simulink model "hyd_hyb_2_opt_cont_test_new_1_col_ef_fin"  (Simulink 7.7)
settings: Solver=ode14x  StartTime=0  StopTime=530  FixedStep=0.01  MaxStep=.4  RelTol=1e-8
InitFcn:
  | const_3
values from neighbouring files (symbols this model uses):
  Af = 6.3    [brk_enrg.m]    (also in brk_enrg_1.m)
  BSFC_906_205 = [3.5684 4.3466 5.1668 6.0769 6.988 7.8992 8.8104 9.7336 10.8548 11.9809 13.1112 14.2571 ... (663 elements, 39x17)]    [BSFC_map_906_205.mat]
  Cd = 0.55    [brk_enrg.m]    (also in brk_enrg_1.m)
  den = 1.202    [brk_enrg.m]    (also in brk_enrg_1.m)
  fr = 0.01    [brk_enrg.m]    (also in brk_enrg_1.m)
undefined symbols (not defined in the file or in its folder): clutchRise, down_spd_2, down_spd_3, down_spd_4, down_spd_c, fuel_density, gearshift, I_wheel, Idle_spd_eng_906, M1_hydr, p_v_15, pmax_125, qv_125, Rw, sec_eng_sfc_map, T_max_906, T_min, TC_spd_ratio_max, torque_convertor, Twait, up_spd_1, up_spd_2, up_spd_3, up_spd_c, v_p_10, v_p_15, v_p_5
libraries: neural x327, fl_lib x43, nesl_utility x30, sdl_lib x14, simulink x4, simulink_need_slupdate x1
(part 3 of 10)

== system hyd_hyb_2_opt_cont_test_new_1_col_ef_fin/Transmission1/Torque Convertor/main solver/Torque generation ==
  note: TORQUE CONVERTER
  note: Not motoring mode is neglected
  Turbine speed (rad/s) : Inport
  Impeller speed (rad/s) : Inport  Port=2
  4 : Product  Inputs=/*  SaturateOnIntegerOverflow=on  RndMeth=Zero  InputSameDT=on  OutDataTypeStr=Inherit: Same as first input
  Constant1 : Constant
  Constant2 : Constant  Value=eps
  Constant6 : Constant  Value=TC_spd_ratio_max
  Gain1 : Gain  Gain=-1  SaturateOnIntegerOverflow=on  OutDataTypeStr=Inherit: Same as input  ParamDataTypeStr=Inherit: Same as input
  Math Function1 : Math  Operator=square  SaturateOnIntegerOverflow=on
  Memory : Memory
  Memory1 : Memory
  MinMax2 : MinMax  Function=max  Inputs=2  ZeroCross=off
  Mu : Lookup  InputValues=torque_convertor(:,1)  Table=torque_convertor(:,2)  SaturateOnIntegerOverflow=on
  Ref_spd (rpm) : Constant  Value=1000
  T1 : Scope  NumInputPorts=2
      settings: YMin=75~-5  YMax=165~5  SaveName=ScopeData19
  T_i : Product  Inputs=**  SaturateOnIntegerOverflow=on  RndMeth=Zero  InputSameDT=on  OutDataTypeStr=Inherit: Same as first input
  T_t : Product  Inputs=**  SaturateOnIntegerOverflow=on  RndMeth=Zero  InputSameDT=on  OutDataTypeStr=Inherit: Same as first input
  check pump spd=0 : Switch  Threshold=0.1
  check turb spd=0 : Switch  Threshold=0.1
  pump T : Lookup  InputValues=torque_convertor(:,1)  Table=torque_convertor(:,3)  SaturateOnIntegerOverflow=on
  rad/s 2 rpm : Gain  Gain=60/(2*pi)
  speed ratio : Product  Inputs=/*  SaturateOnIntegerOverflow=on  RndMeth=Zero  InputSameDT=on  OutDataTypeStr=Inherit: Same as first input
  Turbine torque : Outport
  Impeller torque : Outport  Port=2
  wires:
  Constant2/1 -> MinMax2/2
  MinMax2/1 -> speed ratio/1
  Impeller speed (rad/s)/1 -> MinMax2/1, check pump spd=0/2, rad/s 2 rpm/1
  Turbine speed (rad/s)/1 -> check turb spd=0/2, speed ratio/2
  speed ratio/1 -> check pump spd=0/1
  Constant1/1 -> check turb spd=0/3
  Constant6/1 -> check turb spd=0/1
  check turb spd=0/1 -> check pump spd=0/3
  check pump spd=0/1 -> Mu/1, pump T/1
  Ref_spd (rpm)/1 -> 4/1
  rad/s 2 rpm/1 -> 4/2
  4/1 -> Math Function1/1
  pump T/1 -> T_i/1
  Math Function1/1 -> T_i/2
  T_i/1 -> T_t/2, Gain1/1
  Gain1/1 -> Memory1/1
  Mu/1 -> T_t/1
  T_t/1 -> Memory/1
  Memory/1 -> Turbine torque/1
  Memory1/1 -> Impeller torque/1

== system hyd_hyb_2_opt_cont_test_new_1_col_ef_fin/Transmission1/gear box/gear box/Clutch Control ==
  control : Inport
  1 : Constant
  2 : Constant  Value=2
  3 : Constant  Value=3
  4 : Constant  Value=4
  Add{,1..3} (4 alike) : Sum  Inputs=+-
  Enabled Subsystem1 : Subsystem  TreatAsAtomicUnit=on
  Enabled Subsystem2 : Subsystem  TreatAsAtomicUnit=on
  Enabled Subsystem3 : Subsystem  TreatAsAtomicUnit=on
  Enabled Subsystem4 : Subsystem  TreatAsAtomicUnit=on
  Mux2 : Mux
  disengahe : Constant  Value=-1
  engage : Constant
  selector{1..4} (4 alike) : Switch  Criteria=u2 ~= 0  Threshold=2300  ZeroCross=off
  Clutches : Outport
  wires:
  Mux2/1 -> Clutches/1
  engage/1 -> [engage]
  [disengage] -> selector1/1
  disengahe/1 -> [disengage]
  [engage] -> selector1/3
  control/1 -> Add/1, Add1/1, Add2/1, Add3/1
  Add/1 -> selector1/2
  1/1 -> Add/2
  [disengage] -> selector2/1
  [engage] -> selector2/3
  Add1/1 -> selector2/2
  2/1 -> Add1/2
  [disengage] -> selector3/1
  [engage] -> selector3/3
  Add2/1 -> selector3/2
  3/1 -> Add2/2
  [disengage] -> selector4/1
  [engage] -> selector4/3
  Add3/1 -> selector4/2
  4/1 -> Add3/2
  selector1/1 -> Enabled Subsystem1/Enable
  selector2/1 -> Enabled Subsystem2/Enable
  selector3/1 -> Enabled Subsystem3/Enable
  selector4/1 -> Enabled Subsystem4/Enable
  Enabled Subsystem1/1(clutch release) -> Mux2/1
  Enabled Subsystem2/1(clutch release) -> Mux2/2
  Enabled Subsystem3/1(clutch release) -> Mux2/3
  Enabled Subsystem4/1(clutch release) -> Mux2/4

== system hyd_hyb_2_opt_cont_test_new_1_col_ef_fin/controller1/optimized controller - pm/net_col_ef_1/Layer 1 ==
  "p{1}" : Inport  PortDimensions=3
      mask Display: e = 0.06;c1 = [120 230 180]/255;c2 = ([120 230 180]+0)/(256+128);c3 = ([120 230 180]+128)/(256+128);patch([0 1 1 0],[0 0 1 1],c1);patch([0 1 1 1-e 1-e 0+e],[0 0 1 1-e 0+e 0+e],c2);patch([0 0 1 1-e 0+e 0+e],[0 1 1 1-e 1-e 0+e],c3);plot([0 1 1 0 0],[0 0 1 1 0]);
  Delays 1 : Subsystem
      mask Display: e = 0.06;c1 = [120 150 230]/255;c2 = ([120 150 230]+0)/383;c3 = ([120 150 230]+128)/383;patch([0 1 1 0],[0 0 1 1],c1);patch([0 1 1 1-e 1-e 0+e],[0 0 1 1-e 0+e 0+e],c2);patch([0 0 1 1-e 0+e 0+e],[0 1 1 1-e 1-e 0+e],c3);plot([0 1 1 0 0],[0 0 1 1 0]);disp('0');
  "IW{1,1}" : Subsystem
      mask Display: e = 0.06;c1 = [120 150 230]/255;c2 = ([120 150 230]+0)/383;c3 = ([120 150 230]+128)/383;patch([0 1 1 0],[0 0 1 1],c1);patch([0 1 1 1-e 1-e 0+e],[0 0 1 1-e 0+e 0+e],c2);patch([0 0 1 1-e 0+e 0+e],[0 1 1 1-e 1-e 0+e],c3);plot([0 1 1 0 0],[0 0 1 1 0]);disp('W');
  "b{1}" : Constant  Value=[10.272884338164415;10.158388839610668;-8.8137585907009761;-8.6570271257242233;-8.8970383233546322;-8.3732297223932406;-8.2902058826026686;-8.3765329651302221;-8.1601725859937311;7.3878677135191477;5.9137474143171671;6.0189008328843263;-4.7198199500370155;-4.5492439595817009;-3.6590612602413786;-4.0868738376274472;-3.2611974200680032;-2.5669983522012405;2.8521134680955162;-1.9645715433960607;-2.0075702387778405;-2.2689062882637798;1.7944973393296622;-0.60777657516365402;-0.33335423588948843;0.70492263184083259;1.0038561719860595;0.8312957719409716;2.0241730304275114;2.4288729886427602;-1.5051652534112119;-2.9602742871001562;3.5101998859041661;4.4839700583582864;-5.3527641027608928;4.8621496598397966;-4.4065527200098753;5.333150061440934;5.4587754651459868;6.0824002270216777;6.163842184650008;6.5644779762447678;7.0617890841349729;7.5844337833421029;-8.3589611799416907;9.2543399894272227;9.1887230177194503;-8.8917972218632144;10.192523469036553;-10.477571329366949]
      mask Display: e = 0.06;c1 = [120 150 230]/255;c2 = ([120 150 230]+0)/383;c3 = ([120 150 230]+128)/383;patch([0 1 1 0],[0 0 1 1],c1);patch([0 1 1 1-e 1-e 0+e],[0 0 1 1-e 0+e 0+e],c2);patch([0 0 1 1-e 0+e 0+e],[0 1 1 1-e 1-e 0+e],c3);plot([0 1 1 0 0],[0 0 1 1 0]);disp('b');
  logsig : neural/Transfer Functions/logsig  SystemSampleTime=-1
  netsum : Sum  Inputs=2  SaturateOnIntegerOverflow=on  InputSameDT=on  OutDataTypeStr=Inherit: Same as first input
      mask Display: e = 0.06;c1 = [120 150 230]/255;c2 = ([120 150 230]+0)/383;c3 = ([120 150 230]+128)/383;patch([0 1 1 0],[0 0 1 1],c1);patch([0 1 1 1-e 1-e 0+e],[0 0 1 1-e 0+e 0+e],c2);patch([0 0 1 1-e 0+e 0+e],[0 1 1 1-e 1-e 0+e],c3);plot([0 1 1 0 0],[0 0 1 1 0]);disp('+');
  "a{1}" : Outport  InitialOutput=[0;0;0;0;0;0;0;0;0;0;0;0;0;0;0;0;0;0;0;0;0;0;0;0;0;0;0;0;0;0;0;0;0;0;0;0;0;0;0;0;0;0;0;0;0;0;0;0;0;0]
      mask Display: e = 0.06;c1 = [120 230 180]/255;c2 = ([120 230 180]+0)/(256+128);c3 = ([120 230 180]+128)/(256+128);patch([0 1 1 0],[0 0 1 1],c1);patch([0 1 1 1-e 1-e 0+e],[0 0 1 1-e 0+e 0+e],c2);patch([0 0 1 1-e 0+e 0+e],[0 1 1 1-e 1-e 0+e],c3);plot([0 1 1 0 0],[0 0 1 1 0]);
  wires:
  "p{1}"/1 -> Delays 1/1("p{1}")
  Delays 1/1("pd{1,1}") -> "IW{1,1}"/1("pd{1,1}")
  "IW{1,1}"/1("iz{1,1}") -> netsum/1
  "b{1}"/1 -> netsum/2
  netsum/1 -> logsig/1
  logsig/1 -> "a{1}"/1

== system hyd_hyb_2_opt_cont_test_new_1_col_ef_fin/controller1/optimized controller - pm/net_col_ef_1/Layer 2 ==
  "a{1} " : Inport  PortDimensions=50
      mask Display: e = 0.06;c1 = [120 230 180]/255;c2 = ([120 230 180]+0)/(256+128);c3 = ([120 230 180]+128)/(256+128);patch([0 1 1 0],[0 0 1 1],c1);patch([0 1 1 1-e 1-e 0+e],[0 0 1 1-e 0+e 0+e],c2);patch([0 0 1 1-e 0+e 0+e],[0 1 1 1-e 1-e 0+e],c3);plot([0 1 1 0 0],[0 0 1 1 0]);
  Delays 1 : Subsystem
      mask Display: e = 0.06;c1 = [120 150 230]/255;c2 = ([120 150 230]+0)/383;c3 = ([120 150 230]+128)/383;patch([0 1 1 0],[0 0 1 1],c1);patch([0 1 1 1-e 1-e 0+e],[0 0 1 1-e 0+e 0+e],c2);patch([0 0 1 1-e 0+e 0+e],[0 1 1 1-e 1-e 0+e],c3);plot([0 1 1 0 0],[0 0 1 1 0]);disp('0');
  "LW{2,1}" : Subsystem
      mask Display: e = 0.06;c1 = [120 150 230]/255;c2 = ([120 150 230]+0)/383;c3 = ([120 150 230]+128)/383;patch([0 1 1 0],[0 0 1 1],c1);patch([0 1 1 1-e 1-e 0+e],[0 0 1 1-e 0+e 0+e],c2);patch([0 0 1 1-e 0+e 0+e],[0 1 1 1-e 1-e 0+e],c3);plot([0 1 1 0 0],[0 0 1 1 0]);disp('W');
  "b{2}" : Constant  Value=[-1.4746968992061404;6.761460429459289;4.8593062407264256;-2.4434548501711921;2.8014335830561317;-1.2377617866407475;0.60970112347272343;6.0004453403634397;1.5023634362208427;-2.3253426322313246;-5.3357671798553792;2.2138042378012139;-3.2204621848726322;-0.91358517604309897;-4.265772269140677;-0.49547425424668967;2.7481974655284684;2.6522900082012191;-1.450078084740686;5.9357949258451921;-1.1096734624746596;-1.9216781485245211;1.5013570287327187;-3.1725593392467553;0.070873309951381178;1.4583370245475129;-1.380987170740555;-4.9014727609251594;-2.421891114631245;-0.045879446762915062;2.3447338445340051;5.0580315597432879;2.2792762573025591;4.0979703997466634;-0.41868820623327574;0.59156567080418943;1.93176393811276;3.5095523399155435;-3.5434554285500419;3.8577559424144559;0.1840496036646519;0.80556867719655356;-2.1746365989617589;1.7602851911002209;-0.17757596753320681;5.9726215463790888;-4.0530999585525285;4.0472988103686962;7.3387320715217763;-0.86522529377217905]
      mask Display: e = 0.06;c1 = [120 150 230]/255;c2 = ([120 150 230]+0)/383;c3 = ([120 150 230]+128)/383;patch([0 1 1 0],[0 0 1 1],c1);patch([0 1 1 1-e 1-e 0+e],[0 0 1 1-e 0+e 0+e],c2);patch([0 0 1 1-e 0+e 0+e],[0 1 1 1-e 1-e 0+e],c3);plot([0 1 1 0 0],[0 0 1 1 0]);disp('b');
  logsig : neural/Transfer Functions/logsig  SystemSampleTime=-1
  netsum : Sum  Inputs=2  SaturateOnIntegerOverflow=on  InputSameDT=on  OutDataTypeStr=Inherit: Same as first input
      mask Display: e = 0.06;c1 = [120 150 230]/255;c2 = ([120 150 230]+0)/383;c3 = ([120 150 230]+128)/383;patch([0 1 1 0],[0 0 1 1],c1);patch([0 1 1 1-e 1-e 0+e],[0 0 1 1-e 0+e 0+e],c2);patch([0 0 1 1-e 0+e 0+e],[0 1 1 1-e 1-e 0+e],c3);plot([0 1 1 0 0],[0 0 1 1 0]);disp('+');
  "a{2}" : Outport  InitialOutput=[0;0;0;0;0;0;0;0;0;0;0;0;0;0;0;0;0;0;0;0;0;0;0;0;0;0;0;0;0;0;0;0;0;0;0;0;0;0;0;0;0;0;0;0;0;0;0;0;0;0]
      mask Display: e = 0.06;c1 = [120 230 180]/255;c2 = ([120 230 180]+0)/(256+128);c3 = ([120 230 180]+128)/(256+128);patch([0 1 1 0],[0 0 1 1],c1);patch([0 1 1 1-e 1-e 0+e],[0 0 1 1-e 0+e 0+e],c2);patch([0 0 1 1-e 0+e 0+e],[0 1 1 1-e 1-e 0+e],c3);plot([0 1 1 0 0],[0 0 1 1 0]);
  wires:
  "a{1} "/1 -> Delays 1/1("p{2}")
  Delays 1/1("pd{2,1}") -> "LW{2,1}"/1("ad{2,1}")
  "LW{2,1}"/1("lz{2,1}") -> netsum/1
  "b{2}"/1 -> netsum/2
  netsum/1 -> logsig/1
  logsig/1 -> "a{2}"/1

== system hyd_hyb_2_opt_cont_test_new_1_col_ef_fin/controller1/optimized controller - pm/net_col_ef_1/Layer 3 ==
  "a{2} " : Inport  PortDimensions=50
      mask Display: e = 0.06;c1 = [120 230 180]/255;c2 = ([120 230 180]+0)/(256+128);c3 = ([120 230 180]+128)/(256+128);patch([0 1 1 0],[0 0 1 1],c1);patch([0 1 1 1-e 1-e 0+e],[0 0 1 1-e 0+e 0+e],c2);patch([0 0 1 1-e 0+e 0+e],[0 1 1 1-e 1-e 0+e],c3);plot([0 1 1 0 0],[0 0 1 1 0]);
  Delays 1 : Subsystem
      mask Display: e = 0.06;c1 = [120 150 230]/255;c2 = ([120 150 230]+0)/383;c3 = ([120 150 230]+128)/383;patch([0 1 1 0],[0 0 1 1],c1);patch([0 1 1 1-e 1-e 0+e],[0 0 1 1-e 0+e 0+e],c2);patch([0 0 1 1-e 0+e 0+e],[0 1 1 1-e 1-e 0+e],c3);plot([0 1 1 0 0],[0 0 1 1 0]);disp('0');
  "LW{3,2}" : Subsystem
      mask Display: e = 0.06;c1 = [120 150 230]/255;c2 = ([120 150 230]+0)/383;c3 = ([120 150 230]+128)/383;patch([0 1 1 0],[0 0 1 1],c1);patch([0 1 1 1-e 1-e 0+e],[0 0 1 1-e 0+e 0+e],c2);patch([0 0 1 1-e 0+e 0+e],[0 1 1 1-e 1-e 0+e],c3);plot([0 1 1 0 0],[0 0 1 1 0]);disp('W');
  "b{3}" : Constant  Value=-0.53255115865547076
      mask Display: e = 0.06;c1 = [120 150 230]/255;c2 = ([120 150 230]+0)/383;c3 = ([120 150 230]+128)/383;patch([0 1 1 0],[0 0 1 1],c1);patch([0 1 1 1-e 1-e 0+e],[0 0 1 1-e 0+e 0+e],c2);patch([0 0 1 1-e 0+e 0+e],[0 1 1 1-e 1-e 0+e],c3);plot([0 1 1 0 0],[0 0 1 1 0]);disp('b');
  netsum : Sum  Inputs=2  SaturateOnIntegerOverflow=on  InputSameDT=on  OutDataTypeStr=Inherit: Same as first input
      mask Display: e = 0.06;c1 = [120 150 230]/255;c2 = ([120 150 230]+0)/383;c3 = ([120 150 230]+128)/383;patch([0 1 1 0],[0 0 1 1],c1);patch([0 1 1 1-e 1-e 0+e],[0 0 1 1-e 0+e 0+e],c2);patch([0 0 1 1-e 0+e 0+e],[0 1 1 1-e 1-e 0+e],c3);plot([0 1 1 0 0],[0 0 1 1 0]);disp('+');
  purelin : neural/Transfer Functions/purelin  SystemSampleTime=-1
  "a{3}" : Outport  InitialOutput=0
      mask Display: e = 0.06;c1 = [120 230 180]/255;c2 = ([120 230 180]+0)/(256+128);c3 = ([120 230 180]+128)/(256+128);patch([0 1 1 0],[0 0 1 1],c1);patch([0 1 1 1-e 1-e 0+e],[0 0 1 1-e 0+e 0+e],c2);patch([0 0 1 1-e 0+e 0+e],[0 1 1 1-e 1-e 0+e],c3);plot([0 1 1 0 0],[0 0 1 1 0]);
  wires:
  "a{2} "/1 -> Delays 1/1("p{3}")
  Delays 1/1("pd{3,2}") -> "LW{3,2}"/1("ad{3,2}")
  "LW{3,2}"/1("lz{3,2}") -> netsum/1
  "b{3}"/1 -> netsum/2
  netsum/1 -> purelin/1
  purelin/1 -> "a{3}"/1

== system hyd_hyb_2_opt_cont_test_new_1_col_ef_fin/controller1/optimized controller - pm/net_col_ef_1/Process Input 1 ==
  x : Inport  PortDimensions=3
      mask Display: e = 0.06;c1 = [120 230 180]/255;c2 = ([120 230 180]+0)/(256+128);c3 = ([120 230 180]+128)/(256+128);patch([0 1 1 0],[0 0 1 1],c1);patch([0 1 1 1-e 1-e 0+e],[0 0 1 1-e 0+e 0+e],c2);patch([0 0 1 1-e 0+e 0+e],[0 1 1 1-e 1-e 0+e],c3);plot([0 1 1 0 0],[0 0 1 1 0]);
  fixunknowns : neural/Processing Functions/fixunknowns  SystemSampleTime=-1  inputSize=3  indices=[1 2 3]
  mapminmax : neural/Processing Functions/mapminmax  SystemSampleTime=-1  xmin=[0;0;0]  xmax=[0.90000000000000013;1.009090909090909;0.63716399999999995]  ymin=-1  ymax=1
  removeconstantrows : neural/Processing Functions/removeconstantrows  SystemSampleTime=-1  inputSize=3  keep=[1 2 3]
  p : Outport  PortDimensions=3
      mask Display: e = 0.06;c1 = [120 230 180]/255;c2 = ([120 230 180]+0)/(256+128);c3 = ([120 230 180]+128)/(256+128);patch([0 1 1 0],[0 0 1 1],c1);patch([0 1 1 1-e 1-e 0+e],[0 0 1 1-e 0+e 0+e],c2);patch([0 0 1 1-e 0+e 0+e],[0 1 1 1-e 1-e 0+e],c3);plot([0 1 1 0 0],[0 0 1 1 0]);
  wires:
  x/1 -> fixunknowns/1
  fixunknowns/1 -> removeconstantrows/1
  removeconstantrows/1 -> mapminmax/1
  mapminmax/1 -> p/1

== system hyd_hyb_2_opt_cont_test_new_1_col_ef_fin/controller1/optimized controller - pm/net_col_ef_1/Process Output 1 ==
  a : Inport  PortDimensions=1
      mask Display: e = 0.06;c1 = [120 230 180]/255;c2 = ([120 230 180]+0)/(256+128);c3 = ([120 230 180]+128)/(256+128);patch([0 1 1 0],[0 0 1 1],c1);patch([0 1 1 1-e 1-e 0+e],[0 0 1 1-e 0+e 0+e],c2);patch([0 0 1 1-e 0+e 0+e],[0 1 1 1-e 1-e 0+e],c3);plot([0 1 1 0 0],[0 0 1 1 0]);
  mapminmax_reverse : neural/Processing Functions/mapminmax_reverse  SystemSampleTime=-1  xmin=0  xmax=0.9015181489837879  ymin=-1  ymax=1
  removeconstantrows_reverse : neural/Processing Functions/removeconstantrows_reverse  SystemSampleTime=-1  inputSize=1  constants=zeros(0,1)  rearrange=1
  y : Outport  PortDimensions=1
      mask Display: e = 0.06;c1 = [120 230 180]/255;c2 = ([120 230 180]+0)/(256+128);c3 = ([120 230 180]+128)/(256+128);patch([0 1 1 0],[0 0 1 1],c1);patch([0 1 1 1-e 1-e 0+e],[0 0 1 1-e 0+e 0+e],c2);patch([0 0 1 1-e 0+e 0+e],[0 1 1 1-e 1-e 0+e],c3);plot([0 1 1 0 0],[0 0 1 1 0]);
  wires:
  a/1 -> mapminmax_reverse/1
  mapminmax_reverse/1 -> removeconstantrows_reverse/1
  removeconstantrows_reverse/1 -> y/1

== system hyd_hyb_2_opt_cont_test_new_1_col_ef_fin/controller1/optimized controller - pm/net_col_ef_2/Layer 1 ==
  "p{1}" : Inport  PortDimensions=3
      mask Display: e = 0.06;c1 = [120 230 180]/255;c2 = ([120 230 180]+0)/(256+128);c3 = ([120 230 180]+128)/(256+128);patch([0 1 1 0],[0 0 1 1],c1);patch([0 1 1 1-e 1-e 0+e],[0 0 1 1-e 0+e 0+e],c2);patch([0 0 1 1-e 0+e 0+e],[0 1 1 1-e 1-e 0+e],c3);plot([0 1 1 0 0],[0 0 1 1 0]);
  Delays 1 : Subsystem
      mask Display: e = 0.06;c1 = [120 150 230]/255;c2 = ([120 150 230]+0)/383;c3 = ([120 150 230]+128)/383;patch([0 1 1 0],[0 0 1 1],c1);patch([0 1 1 1-e 1-e 0+e],[0 0 1 1-e 0+e 0+e],c2);patch([0 0 1 1-e 0+e 0+e],[0 1 1 1-e 1-e 0+e],c3);plot([0 1 1 0 0],[0 0 1 1 0]);disp('0');
  "IW{1,1}" : Subsystem
      mask Display: e = 0.06;c1 = [120 150 230]/255;c2 = ([120 150 230]+0)/383;c3 = ([120 150 230]+128)/383;patch([0 1 1 0],[0 0 1 1],c1);patch([0 1 1 1-e 1-e 0+e],[0 0 1 1-e 0+e 0+e],c2);patch([0 0 1 1-e 0+e 0+e],[0 1 1 1-e 1-e 0+e],c3);plot([0 1 1 0 0],[0 0 1 1 0]);disp('W');
  "b{1}" : Constant  Value=[11.06291160506464;9.6569498895400336;9.7057218735701358;9.3112833261288372;8.7376413828696577;7.5818969929168896;-7.689186662963075;6.8841555682455375;5.480543380122934;-6.7353338753925431;-6.2439434769565203;-4.7494739295836874;-4.95737643411577;-4.6437259198738037;3.5304849746771545;-4.1757390830539922;-3.0584729883330146;-3.1420690410497674;-2.7312479968531616;-2.761085247415719;0.94765649190303802;1.1617110605498155;0.97691124339635782;0.79251198170241977;0.20894216666912813;-0.89968169007623477;-0.5079308913259809;-1.1247392235072682;1.7484351351117244;-1.7461420332640352;-2.3679372815024879;-2.4585499737006038;4.5049715514684214;3.7433756567561591;4.3924005740068113;-4.4562245200249722;4.5180694005112034;-5.3308269964363113;5.9176445995746247;-6.1338393655658079;-6.5153465860809519;-6.9387105180769808;8.3926806026615441;-7.8456184342767861;8.170511983096354;8.7628634893332684;-9.0774508782222547;-8.537231421878209;-9.8218508072603683;9.9868721404365726]
      mask Display: e = 0.06;c1 = [120 150 230]/255;c2 = ([120 150 230]+0)/383;c3 = ([120 150 230]+128)/383;patch([0 1 1 0],[0 0 1 1],c1);patch([0 1 1 1-e 1-e 0+e],[0 0 1 1-e 0+e 0+e],c2);patch([0 0 1 1-e 0+e 0+e],[0 1 1 1-e 1-e 0+e],c3);plot([0 1 1 0 0],[0 0 1 1 0]);disp('b');
  logsig : neural/Transfer Functions/logsig  SystemSampleTime=-1
  netsum : Sum  Inputs=2  SaturateOnIntegerOverflow=on  InputSameDT=on  OutDataTypeStr=Inherit: Same as first input
      mask Display: e = 0.06;c1 = [120 150 230]/255;c2 = ([120 150 230]+0)/383;c3 = ([120 150 230]+128)/383;patch([0 1 1 0],[0 0 1 1],c1);patch([0 1 1 1-e 1-e 0+e],[0 0 1 1-e 0+e 0+e],c2);patch([0 0 1 1-e 0+e 0+e],[0 1 1 1-e 1-e 0+e],c3);plot([0 1 1 0 0],[0 0 1 1 0]);disp('+');
  "a{1}" : Outport  InitialOutput=[0;0;0;0;0;0;0;0;0;0;0;0;0;0;0;0;0;0;0;0;0;0;0;0;0;0;0;0;0;0;0;0;0;0;0;0;0;0;0;0;0;0;0;0;0;0;0;0;0;0]
      mask Display: e = 0.06;c1 = [120 230 180]/255;c2 = ([120 230 180]+0)/(256+128);c3 = ([120 230 180]+128)/(256+128);patch([0 1 1 0],[0 0 1 1],c1);patch([0 1 1 1-e 1-e 0+e],[0 0 1 1-e 0+e 0+e],c2);patch([0 0 1 1-e 0+e 0+e],[0 1 1 1-e 1-e 0+e],c3);plot([0 1 1 0 0],[0 0 1 1 0]);
  wires:
  "p{1}"/1 -> Delays 1/1("p{1}")
  Delays 1/1("pd{1,1}") -> "IW{1,1}"/1("pd{1,1}")
  "IW{1,1}"/1("iz{1,1}") -> netsum/1
  "b{1}"/1 -> netsum/2
  netsum/1 -> logsig/1
  logsig/1 -> "a{1}"/1

== system hyd_hyb_2_opt_cont_test_new_1_col_ef_fin/controller1/optimized controller - pm/net_col_ef_2/Layer 2 ==
  "a{1} " : Inport  PortDimensions=50
      mask Display: e = 0.06;c1 = [120 230 180]/255;c2 = ([120 230 180]+0)/(256+128);c3 = ([120 230 180]+128)/(256+128);patch([0 1 1 0],[0 0 1 1],c1);patch([0 1 1 1-e 1-e 0+e],[0 0 1 1-e 0+e 0+e],c2);patch([0 0 1 1-e 0+e 0+e],[0 1 1 1-e 1-e 0+e],c3);plot([0 1 1 0 0],[0 0 1 1 0]);
  Delays 1 : Subsystem
      mask Display: e = 0.06;c1 = [120 150 230]/255;c2 = ([120 150 230]+0)/383;c3 = ([120 150 230]+128)/383;patch([0 1 1 0],[0 0 1 1],c1);patch([0 1 1 1-e 1-e 0+e],[0 0 1 1-e 0+e 0+e],c2);patch([0 0 1 1-e 0+e 0+e],[0 1 1 1-e 1-e 0+e],c3);plot([0 1 1 0 0],[0 0 1 1 0]);disp('0');
  "LW{2,1}" : Subsystem
      mask Display: e = 0.06;c1 = [120 150 230]/255;c2 = ([120 150 230]+0)/383;c3 = ([120 150 230]+128)/383;patch([0 1 1 0],[0 0 1 1],c1);patch([0 1 1 1-e 1-e 0+e],[0 0 1 1-e 0+e 0+e],c2);patch([0 0 1 1-e 0+e 0+e],[0 1 1 1-e 1-e 0+e],c3);plot([0 1 1 0 0],[0 0 1 1 0]);disp('W');
  "b{2}" : Constant  Value=[1.2957023881188001;-8.4250423006678865;-0.83849144117593744;5.1940231045960283;-2.8277581624328021;2.323521888729871;-0.47657758453361571;-1.4935523337583885;6.2630674201555294;3.9356633739489526;-3.3711843755045723;-0.91849200872177161;2.3155313979295107;5.2316800014222249;-1.549962088505253;2.6578906811948371;-4.0210651554100005;1.1726109689860429;-3.5551891275712766;-0.63513021573007333;0.78168202695753253;-2.5466977416139245;-3.1494465602922777;4.5806898083337355;7.8804370668016537;2.0015927562451705;4.4640169205076878;-0.85047345033081234;4.2406992651338431;-4.5935384604573288;-3.278093976124933;-4.5782806163281355;-1.363012863764252;-0.91938331656109173;-4.9024295612468514;0.8809270622210823;-0.66333942549327818;-0.49112451411523284;-5.6624444398120888;-0.84647761333632732;-2.5444084615881972;-8.0610468494463348;0.61998104669407039;-4.5620258732554246;0.45894670318714587;1.1974781726729835;2.2804204429841644;0.38514422559041417;2.8834613502054052;-0.82401605208817619]
      mask Display: e = 0.06;c1 = [120 150 230]/255;c2 = ([120 150 230]+0)/383;c3 = ([120 150 230]+128)/383;patch([0 1 1 0],[0 0 1 1],c1);patch([0 1 1 1-e 1-e 0+e],[0 0 1 1-e 0+e 0+e],c2);patch([0 0 1 1-e 0+e 0+e],[0 1 1 1-e 1-e 0+e],c3);plot([0 1 1 0 0],[0 0 1 1 0]);disp('b');
  logsig : neural/Transfer Functions/logsig  SystemSampleTime=-1
  netsum : Sum  Inputs=2  SaturateOnIntegerOverflow=on  InputSameDT=on  OutDataTypeStr=Inherit: Same as first input
      mask Display: e = 0.06;c1 = [120 150 230]/255;c2 = ([120 150 230]+0)/383;c3 = ([120 150 230]+128)/383;patch([0 1 1 0],[0 0 1 1],c1);patch([0 1 1 1-e 1-e 0+e],[0 0 1 1-e 0+e 0+e],c2);patch([0 0 1 1-e 0+e 0+e],[0 1 1 1-e 1-e 0+e],c3);plot([0 1 1 0 0],[0 0 1 1 0]);disp('+');
  "a{2}" : Outport  InitialOutput=[0;0;0;0;0;0;0;0;0;0;0;0;0;0;0;0;0;0;0;0;0;0;0;0;0;0;0;0;0;0;0;0;0;0;0;0;0;0;0;0;0;0;0;0;0;0;0;0;0;0]
      mask Display: e = 0.06;c1 = [120 230 180]/255;c2 = ([120 230 180]+0)/(256+128);c3 = ([120 230 180]+128)/(256+128);patch([0 1 1 0],[0 0 1 1],c1);patch([0 1 1 1-e 1-e 0+e],[0 0 1 1-e 0+e 0+e],c2);patch([0 0 1 1-e 0+e 0+e],[0 1 1 1-e 1-e 0+e],c3);plot([0 1 1 0 0],[0 0 1 1 0]);
  wires:
  "a{1} "/1 -> Delays 1/1("p{2}")
  Delays 1/1("pd{2,1}") -> "LW{2,1}"/1("ad{2,1}")
  "LW{2,1}"/1("lz{2,1}") -> netsum/1
  "b{2}"/1 -> netsum/2
  netsum/1 -> logsig/1
  logsig/1 -> "a{2}"/1

== system hyd_hyb_2_opt_cont_test_new_1_col_ef_fin/controller1/optimized controller - pm/net_col_ef_2/Layer 3 ==
  "a{2} " : Inport  PortDimensions=50
      mask Display: e = 0.06;c1 = [120 230 180]/255;c2 = ([120 230 180]+0)/(256+128);c3 = ([120 230 180]+128)/(256+128);patch([0 1 1 0],[0 0 1 1],c1);patch([0 1 1 1-e 1-e 0+e],[0 0 1 1-e 0+e 0+e],c2);patch([0 0 1 1-e 0+e 0+e],[0 1 1 1-e 1-e 0+e],c3);plot([0 1 1 0 0],[0 0 1 1 0]);
  Delays 1 : Subsystem
      mask Display: e = 0.06;c1 = [120 150 230]/255;c2 = ([120 150 230]+0)/383;c3 = ([120 150 230]+128)/383;patch([0 1 1 0],[0 0 1 1],c1);patch([0 1 1 1-e 1-e 0+e],[0 0 1 1-e 0+e 0+e],c2);patch([0 0 1 1-e 0+e 0+e],[0 1 1 1-e 1-e 0+e],c3);plot([0 1 1 0 0],[0 0 1 1 0]);disp('0');
  "LW{3,2}" : Subsystem
      mask Display: e = 0.06;c1 = [120 150 230]/255;c2 = ([120 150 230]+0)/383;c3 = ([120 150 230]+128)/383;patch([0 1 1 0],[0 0 1 1],c1);patch([0 1 1 1-e 1-e 0+e],[0 0 1 1-e 0+e 0+e],c2);patch([0 0 1 1-e 0+e 0+e],[0 1 1 1-e 1-e 0+e],c3);plot([0 1 1 0 0],[0 0 1 1 0]);disp('W');
  "b{3}" : Constant  Value=0.26564128559593225
      mask Display: e = 0.06;c1 = [120 150 230]/255;c2 = ([120 150 230]+0)/383;c3 = ([120 150 230]+128)/383;patch([0 1 1 0],[0 0 1 1],c1);patch([0 1 1 1-e 1-e 0+e],[0 0 1 1-e 0+e 0+e],c2);patch([0 0 1 1-e 0+e 0+e],[0 1 1 1-e 1-e 0+e],c3);plot([0 1 1 0 0],[0 0 1 1 0]);disp('b');
  netsum : Sum  Inputs=2  SaturateOnIntegerOverflow=on  InputSameDT=on  OutDataTypeStr=Inherit: Same as first input
      mask Display: e = 0.06;c1 = [120 150 230]/255;c2 = ([120 150 230]+0)/383;c3 = ([120 150 230]+128)/383;patch([0 1 1 0],[0 0 1 1],c1);patch([0 1 1 1-e 1-e 0+e],[0 0 1 1-e 0+e 0+e],c2);patch([0 0 1 1-e 0+e 0+e],[0 1 1 1-e 1-e 0+e],c3);plot([0 1 1 0 0],[0 0 1 1 0]);disp('+');
  purelin : neural/Transfer Functions/purelin  SystemSampleTime=-1
  "a{3}" : Outport  InitialOutput=0
      mask Display: e = 0.06;c1 = [120 230 180]/255;c2 = ([120 230 180]+0)/(256+128);c3 = ([120 230 180]+128)/(256+128);patch([0 1 1 0],[0 0 1 1],c1);patch([0 1 1 1-e 1-e 0+e],[0 0 1 1-e 0+e 0+e],c2);patch([0 0 1 1-e 0+e 0+e],[0 1 1 1-e 1-e 0+e],c3);plot([0 1 1 0 0],[0 0 1 1 0]);
  wires:
  "a{2} "/1 -> Delays 1/1("p{3}")
  Delays 1/1("pd{3,2}") -> "LW{3,2}"/1("ad{3,2}")
  "LW{3,2}"/1("lz{3,2}") -> netsum/1
  "b{3}"/1 -> netsum/2
  netsum/1 -> purelin/1
  purelin/1 -> "a{3}"/1

== system hyd_hyb_2_opt_cont_test_new_1_col_ef_fin/controller1/optimized controller - pm/net_col_ef_2/Process Input 1 ==
  x : Inport  PortDimensions=3
      mask Display: e = 0.06;c1 = [120 230 180]/255;c2 = ([120 230 180]+0)/(256+128);c3 = ([120 230 180]+128)/(256+128);patch([0 1 1 0],[0 0 1 1],c1);patch([0 1 1 1-e 1-e 0+e],[0 0 1 1-e 0+e 0+e],c2);patch([0 0 1 1-e 0+e 0+e],[0 1 1 1-e 1-e 0+e],c3);plot([0 1 1 0 0],[0 0 1 1 0]);
  fixunknowns : neural/Processing Functions/fixunknowns  SystemSampleTime=-1  inputSize=3  indices=[1 2 3]
  mapminmax : neural/Processing Functions/mapminmax  SystemSampleTime=-1  xmin=[0;-1;0]  xmax=[0.90000000000000013;0;0.60176599999999991]  ymin=-1  ymax=1
  removeconstantrows : neural/Processing Functions/removeconstantrows  SystemSampleTime=-1  inputSize=3  keep=[1 2 3]
  p : Outport  PortDimensions=3
      mask Display: e = 0.06;c1 = [120 230 180]/255;c2 = ([120 230 180]+0)/(256+128);c3 = ([120 230 180]+128)/(256+128);patch([0 1 1 0],[0 0 1 1],c1);patch([0 1 1 1-e 1-e 0+e],[0 0 1 1-e 0+e 0+e],c2);patch([0 0 1 1-e 0+e 0+e],[0 1 1 1-e 1-e 0+e],c3);plot([0 1 1 0 0],[0 0 1 1 0]);
  wires:
  x/1 -> fixunknowns/1
  fixunknowns/1 -> removeconstantrows/1
  removeconstantrows/1 -> mapminmax/1
  mapminmax/1 -> p/1

== system hyd_hyb_2_opt_cont_test_new_1_col_ef_fin/controller1/optimized controller - pm/net_col_ef_2/Process Output 1 ==
  a : Inport  PortDimensions=1
      mask Display: e = 0.06;c1 = [120 230 180]/255;c2 = ([120 230 180]+0)/(256+128);c3 = ([120 230 180]+128)/(256+128);patch([0 1 1 0],[0 0 1 1],c1);patch([0 1 1 1-e 1-e 0+e],[0 0 1 1-e 0+e 0+e],c2);patch([0 0 1 1-e 0+e 0+e],[0 1 1 1-e 1-e 0+e],c3);plot([0 1 1 0 0],[0 0 1 1 0]);
  mapminmax_reverse : neural/Processing Functions/mapminmax_reverse  SystemSampleTime=-1  xmin=-0.82656534503385148  xmax=0  ymin=-1  ymax=1
  removeconstantrows_reverse : neural/Processing Functions/removeconstantrows_reverse  SystemSampleTime=-1  inputSize=1  constants=zeros(0,1)  rearrange=1
  y : Outport  PortDimensions=1
      mask Display: e = 0.06;c1 = [120 230 180]/255;c2 = ([120 230 180]+0)/(256+128);c3 = ([120 230 180]+128)/(256+128);patch([0 1 1 0],[0 0 1 1],c1);patch([0 1 1 1-e 1-e 0+e],[0 0 1 1-e 0+e 0+e],c2);patch([0 0 1 1-e 0+e 0+e],[0 1 1 1-e 1-e 0+e],c3);plot([0 1 1 0 0],[0 0 1 1 0]);
  wires:
  a/1 -> mapminmax_reverse/1
  mapminmax_reverse/1 -> removeconstantrows_reverse/1
  removeconstantrows_reverse/1 -> y/1

== system hyd_hyb_2_opt_cont_test_new_1_col_ef_fin/controller1/optimized controller - pm1/net_col_ef_3/Layer 1 ==
  "p{1}" : Inport  PortDimensions=3
      mask Display: e = 0.06;c1 = [120 230 180]/255;c2 = ([120 230 180]+0)/(256+128);c3 = ([120 230 180]+128)/(256+128);patch([0 1 1 0],[0 0 1 1],c1);patch([0 1 1 1-e 1-e 0+e],[0 0 1 1-e 0+e 0+e],c2);patch([0 0 1 1-e 0+e 0+e],[0 1 1 1-e 1-e 0+e],c3);plot([0 1 1 0 0],[0 0 1 1 0]);
  Delays 1 : Subsystem
      mask Display: e = 0.06;c1 = [120 150 230]/255;c2 = ([120 150 230]+0)/383;c3 = ([120 150 230]+128)/383;patch([0 1 1 0],[0 0 1 1],c1);patch([0 1 1 1-e 1-e 0+e],[0 0 1 1-e 0+e 0+e],c2);patch([0 0 1 1-e 0+e 0+e],[0 1 1 1-e 1-e 0+e],c3);plot([0 1 1 0 0],[0 0 1 1 0]);disp('0');
  "IW{1,1}" : Subsystem
      mask Display: e = 0.06;c1 = [120 150 230]/255;c2 = ([120 150 230]+0)/383;c3 = ([120 150 230]+128)/383;patch([0 1 1 0],[0 0 1 1],c1);patch([0 1 1 1-e 1-e 0+e],[0 0 1 1-e 0+e 0+e],c2);patch([0 0 1 1-e 0+e 0+e],[0 1 1 1-e 1-e 0+e],c3);plot([0 1 1 0 0],[0 0 1 1 0]);disp('W');
  "b{1}" : Constant  Value=[-10.643683230191794;-10.229055835795645;-9.8419361586136098;8.9292071904240498;-7.9301200498881341;-8.5312276367166398;-8.0787332817090807;-7.1801829651784956;-7.1422979669895925;7.6574507400526244;-6.8058320866776443;5.7726303938873196;5.0942577326902718;-4.4190742266869023;-4.2000050539414406;3.3156844915441188;-3.6018330315902674;3.2111340201154821;3.4063231399051173;2.713673686793284;-2.2969262000323476;-0.95798194486405619;1.3882428678065137;0.53274842174130221;0.35161112190908794;-0.53305901979814652;-0.31544532796981212;0.75612601374056487;1.6943613795083348;1.9759736633342488;-1.7730161980491879;2.509319885314572;-3.594923701995707;-3.3778535798122959;3.9191871128199467;-4.4281133880481089;4.7810609741816759;5.0406994158902352;5.4501704751636275;-6.0616240519998943;-6.4444625714767829;7.0634843414245951;-7.4313377140042371;-7.8215993589828736;-8.2106177232952007;-9.0008353434187995;-9.1001035805791375;9.5079395238110305;-9.8813983709672435;-10.024804110235156]
      mask Display: e = 0.06;c1 = [120 150 230]/255;c2 = ([120 150 230]+0)/383;c3 = ([120 150 230]+128)/383;patch([0 1 1 0],[0 0 1 1],c1);patch([0 1 1 1-e 1-e 0+e],[0 0 1 1-e 0+e 0+e],c2);patch([0 0 1 1-e 0+e 0+e],[0 1 1 1-e 1-e 0+e],c3);plot([0 1 1 0 0],[0 0 1 1 0]);disp('b');
  logsig : neural/Transfer Functions/logsig  SystemSampleTime=-1
  netsum : Sum  Inputs=2  SaturateOnIntegerOverflow=on  InputSameDT=on  OutDataTypeStr=Inherit: Same as first input
      mask Display: e = 0.06;c1 = [120 150 230]/255;c2 = ([120 150 230]+0)/383;c3 = ([120 150 230]+128)/383;patch([0 1 1 0],[0 0 1 1],c1);patch([0 1 1 1-e 1-e 0+e],[0 0 1 1-e 0+e 0+e],c2);patch([0 0 1 1-e 0+e 0+e],[0 1 1 1-e 1-e 0+e],c3);plot([0 1 1 0 0],[0 0 1 1 0]);disp('+');
  "a{1}" : Outport  InitialOutput=[0;0;0;0;0;0;0;0;0;0;0;0;0;0;0;0;0;0;0;0;0;0;0;0;0;0;0;0;0;0;0;0;0;0;0;0;0;0;0;0;0;0;0;0;0;0;0;0;0;0]
      mask Display: e = 0.06;c1 = [120 230 180]/255;c2 = ([120 230 180]+0)/(256+128);c3 = ([120 230 180]+128)/(256+128);patch([0 1 1 0],[0 0 1 1],c1);patch([0 1 1 1-e 1-e 0+e],[0 0 1 1-e 0+e 0+e],c2);patch([0 0 1 1-e 0+e 0+e],[0 1 1 1-e 1-e 0+e],c3);plot([0 1 1 0 0],[0 0 1 1 0]);
  wires:
  "p{1}"/1 -> Delays 1/1("p{1}")
  Delays 1/1("pd{1,1}") -> "IW{1,1}"/1("pd{1,1}")
  "IW{1,1}"/1("iz{1,1}") -> netsum/1
  "b{1}"/1 -> netsum/2
  netsum/1 -> logsig/1
  logsig/1 -> "a{1}"/1

== system hyd_hyb_2_opt_cont_test_new_1_col_ef_fin/controller1/optimized controller - pm1/net_col_ef_3/Layer 2 ==
  "a{1} " : Inport  PortDimensions=50
      mask Display: e = 0.06;c1 = [120 230 180]/255;c2 = ([120 230 180]+0)/(256+128);c3 = ([120 230 180]+128)/(256+128);patch([0 1 1 0],[0 0 1 1],c1);patch([0 1 1 1-e 1-e 0+e],[0 0 1 1-e 0+e 0+e],c2);patch([0 0 1 1-e 0+e 0+e],[0 1 1 1-e 1-e 0+e],c3);plot([0 1 1 0 0],[0 0 1 1 0]);
  Delays 1 : Subsystem
      mask Display: e = 0.06;c1 = [120 150 230]/255;c2 = ([120 150 230]+0)/383;c3 = ([120 150 230]+128)/383;patch([0 1 1 0],[0 0 1 1],c1);patch([0 1 1 1-e 1-e 0+e],[0 0 1 1-e 0+e 0+e],c2);patch([0 0 1 1-e 0+e 0+e],[0 1 1 1-e 1-e 0+e],c3);plot([0 1 1 0 0],[0 0 1 1 0]);disp('0');
  "LW{2,1}" : Subsystem
      mask Display: e = 0.06;c1 = [120 150 230]/255;c2 = ([120 150 230]+0)/383;c3 = ([120 150 230]+128)/383;patch([0 1 1 0],[0 0 1 1],c1);patch([0 1 1 1-e 1-e 0+e],[0 0 1 1-e 0+e 0+e],c2);patch([0 0 1 1-e 0+e 0+e],[0 1 1 1-e 1-e 0+e],c3);plot([0 1 1 0 0],[0 0 1 1 0]);disp('W');
  "b{2}" : Constant  Value=[0.33265670861233171;6.1680935912721031;6.1199868543859894;7.8131837218514137;3.9834389911107131;-0.60925756290193422;-7.8310898747422657;-3.8497726038614624;-10.518914257631145;4.6208002186091202;-5.6308581980076502;-1.9542990342777016;6.4201576427938534;-1.465910595845314;-1.7392360119725558;-2.3672205297193041;2.434787958609653;1.8513305210833275;1.8063049578172605;0.0082909993322452628;2.2766223703787123;2.1396423088487659;0.11180475182179944;-5.4987680582330514;0.08150224079792466;-4.5162938193899942;2.479300547137564;3.4062158491394698;7.873120614301599;3.7256297792501165;-2.4857044245850082;4.1861509399074412;-0.78905391228865773;3.0119595137994182;0.32853262304526698;2.1291363091449087;-3.7753097503260045;2.3464033284223058;-0.70605462945011754;1.9116106002930648;0.98107913780429001;-2.1273684428658157;2.5567302624895563;10.549746977836262;-6.3611311430471744;-5.429841703571979;-3.8482631426718252;-4.1664577165241026;1.5237682737593172;4.6928752478698366]
      mask Display: e = 0.06;c1 = [120 150 230]/255;c2 = ([120 150 230]+0)/383;c3 = ([120 150 230]+128)/383;patch([0 1 1 0],[0 0 1 1],c1);patch([0 1 1 1-e 1-e 0+e],[0 0 1 1-e 0+e 0+e],c2);patch([0 0 1 1-e 0+e 0+e],[0 1 1 1-e 1-e 0+e],c3);plot([0 1 1 0 0],[0 0 1 1 0]);disp('b');
  logsig : neural/Transfer Functions/logsig  SystemSampleTime=-1
  netsum : Sum  Inputs=2  SaturateOnIntegerOverflow=on  InputSameDT=on  OutDataTypeStr=Inherit: Same as first input
      mask Display: e = 0.06;c1 = [120 150 230]/255;c2 = ([120 150 230]+0)/383;c3 = ([120 150 230]+128)/383;patch([0 1 1 0],[0 0 1 1],c1);patch([0 1 1 1-e 1-e 0+e],[0 0 1 1-e 0+e 0+e],c2);patch([0 0 1 1-e 0+e 0+e],[0 1 1 1-e 1-e 0+e],c3);plot([0 1 1 0 0],[0 0 1 1 0]);disp('+');
  "a{2}" : Outport  InitialOutput=[0;0;0;0;0;0;0;0;0;0;0;0;0;0;0;0;0;0;0;0;0;0;0;0;0;0;0;0;0;0;0;0;0;0;0;0;0;0;0;0;0;0;0;0;0;0;0;0;0;0]
      mask Display: e = 0.06;c1 = [120 230 180]/255;c2 = ([120 230 180]+0)/(256+128);c3 = ([120 230 180]+128)/(256+128);patch([0 1 1 0],[0 0 1 1],c1);patch([0 1 1 1-e 1-e 0+e],[0 0 1 1-e 0+e 0+e],c2);patch([0 0 1 1-e 0+e 0+e],[0 1 1 1-e 1-e 0+e],c3);plot([0 1 1 0 0],[0 0 1 1 0]);
  wires:
  "a{1} "/1 -> Delays 1/1("p{2}")
  Delays 1/1("pd{2,1}") -> "LW{2,1}"/1("ad{2,1}")
  "LW{2,1}"/1("lz{2,1}") -> netsum/1
  "b{2}"/1 -> netsum/2
  netsum/1 -> logsig/1
  logsig/1 -> "a{2}"/1

== system hyd_hyb_2_opt_cont_test_new_1_col_ef_fin/controller1/optimized controller - pm1/net_col_ef_3/Layer 3 ==
  "a{2} " : Inport  PortDimensions=50
      mask Display: e = 0.06;c1 = [120 230 180]/255;c2 = ([120 230 180]+0)/(256+128);c3 = ([120 230 180]+128)/(256+128);patch([0 1 1 0],[0 0 1 1],c1);patch([0 1 1 1-e 1-e 0+e],[0 0 1 1-e 0+e 0+e],c2);patch([0 0 1 1-e 0+e 0+e],[0 1 1 1-e 1-e 0+e],c3);plot([0 1 1 0 0],[0 0 1 1 0]);
  Delays 1 : Subsystem
      mask Display: e = 0.06;c1 = [120 150 230]/255;c2 = ([120 150 230]+0)/383;c3 = ([120 150 230]+128)/383;patch([0 1 1 0],[0 0 1 1],c1);patch([0 1 1 1-e 1-e 0+e],[0 0 1 1-e 0+e 0+e],c2);patch([0 0 1 1-e 0+e 0+e],[0 1 1 1-e 1-e 0+e],c3);plot([0 1 1 0 0],[0 0 1 1 0]);disp('0');
  "LW{3,2}" : Subsystem
      mask Display: e = 0.06;c1 = [120 150 230]/255;c2 = ([120 150 230]+0)/383;c3 = ([120 150 230]+128)/383;patch([0 1 1 0],[0 0 1 1],c1);patch([0 1 1 1-e 1-e 0+e],[0 0 1 1-e 0+e 0+e],c2);patch([0 0 1 1-e 0+e 0+e],[0 1 1 1-e 1-e 0+e],c3);plot([0 1 1 0 0],[0 0 1 1 0]);disp('W');
  "b{3}" : Constant  Value=-0.12041582034577576
      mask Display: e = 0.06;c1 = [120 150 230]/255;c2 = ([120 150 230]+0)/383;c3 = ([120 150 230]+128)/383;patch([0 1 1 0],[0 0 1 1],c1);patch([0 1 1 1-e 1-e 0+e],[0 0 1 1-e 0+e 0+e],c2);patch([0 0 1 1-e 0+e 0+e],[0 1 1 1-e 1-e 0+e],c3);plot([0 1 1 0 0],[0 0 1 1 0]);disp('b');
  netsum : Sum  Inputs=2  SaturateOnIntegerOverflow=on  InputSameDT=on  OutDataTypeStr=Inherit: Same as first input
      mask Display: e = 0.06;c1 = [120 150 230]/255;c2 = ([120 150 230]+0)/383;c3 = ([120 150 230]+128)/383;patch([0 1 1 0],[0 0 1 1],c1);patch([0 1 1 1-e 1-e 0+e],[0 0 1 1-e 0+e 0+e],c2);patch([0 0 1 1-e 0+e 0+e],[0 1 1 1-e 1-e 0+e],c3);plot([0 1 1 0 0],[0 0 1 1 0]);disp('+');
  purelin : neural/Transfer Functions/purelin  SystemSampleTime=-1
  "a{3}" : Outport  InitialOutput=0
      mask Display: e = 0.06;c1 = [120 230 180]/255;c2 = ([120 230 180]+0)/(256+128);c3 = ([120 230 180]+128)/(256+128);patch([0 1 1 0],[0 0 1 1],c1);patch([0 1 1 1-e 1-e 0+e],[0 0 1 1-e 0+e 0+e],c2);patch([0 0 1 1-e 0+e 0+e],[0 1 1 1-e 1-e 0+e],c3);plot([0 1 1 0 0],[0 0 1 1 0]);
  wires:
  "a{2} "/1 -> Delays 1/1("p{3}")
  Delays 1/1("pd{3,2}") -> "LW{3,2}"/1("ad{3,2}")
  "LW{3,2}"/1("lz{3,2}") -> netsum/1
  "b{3}"/1 -> netsum/2
  netsum/1 -> purelin/1
  purelin/1 -> "a{3}"/1

== system hyd_hyb_2_opt_cont_test_new_1_col_ef_fin/controller1/optimized controller - pm1/net_col_ef_3/Process Input 1 ==
  x : Inport  PortDimensions=3
      mask Display: e = 0.06;c1 = [120 230 180]/255;c2 = ([120 230 180]+0)/(256+128);c3 = ([120 230 180]+128)/(256+128);patch([0 1 1 0],[0 0 1 1],c1);patch([0 1 1 1-e 1-e 0+e],[0 0 1 1-e 0+e 0+e],c2);patch([0 0 1 1-e 0+e 0+e],[0 1 1 1-e 1-e 0+e],c3);plot([0 1 1 0 0],[0 0 1 1 0]);
  fixunknowns : neural/Processing Functions/fixunknowns  SystemSampleTime=-1  inputSize=3  indices=[1 2 3]
  mapminmax : neural/Processing Functions/mapminmax  SystemSampleTime=-1  xmin=[0;0;0]  xmax=[0.90000000000000013;1.009090909090909;0.63716399999999995]  ymin=-1  ymax=1
  removeconstantrows : neural/Processing Functions/removeconstantrows  SystemSampleTime=-1  inputSize=3  keep=[1 2 3]
  p : Outport  PortDimensions=3
      mask Display: e = 0.06;c1 = [120 230 180]/255;c2 = ([120 230 180]+0)/(256+128);c3 = ([120 230 180]+128)/(256+128);patch([0 1 1 0],[0 0 1 1],c1);patch([0 1 1 1-e 1-e 0+e],[0 0 1 1-e 0+e 0+e],c2);patch([0 0 1 1-e 0+e 0+e],[0 1 1 1-e 1-e 0+e],c3);plot([0 1 1 0 0],[0 0 1 1 0]);
  wires:
  x/1 -> fixunknowns/1
  fixunknowns/1 -> removeconstantrows/1
  removeconstantrows/1 -> mapminmax/1
  mapminmax/1 -> p/1

== system hyd_hyb_2_opt_cont_test_new_1_col_ef_fin/controller1/optimized controller - pm1/net_col_ef_3/Process Output 1 ==
  a : Inport  PortDimensions=1
      mask Display: e = 0.06;c1 = [120 230 180]/255;c2 = ([120 230 180]+0)/(256+128);c3 = ([120 230 180]+128)/(256+128);patch([0 1 1 0],[0 0 1 1],c1);patch([0 1 1 1-e 1-e 0+e],[0 0 1 1-e 0+e 0+e],c2);patch([0 0 1 1-e 0+e 0+e],[0 1 1 1-e 1-e 0+e],c3);plot([0 1 1 0 0],[0 0 1 1 0]);
  mapminmax_reverse : neural/Processing Functions/mapminmax_reverse  SystemSampleTime=-1  xmin=0  xmax=1.009090909090909  ymin=-1  ymax=1
  removeconstantrows_reverse : neural/Processing Functions/removeconstantrows_reverse  SystemSampleTime=-1  inputSize=1  constants=zeros(0,1)  rearrange=1
  y : Outport  PortDimensions=1
      mask Display: e = 0.06;c1 = [120 230 180]/255;c2 = ([120 230 180]+0)/(256+128);c3 = ([120 230 180]+128)/(256+128);patch([0 1 1 0],[0 0 1 1],c1);patch([0 1 1 1-e 1-e 0+e],[0 0 1 1-e 0+e 0+e],c2);patch([0 0 1 1-e 0+e 0+e],[0 1 1 1-e 1-e 0+e],c3);plot([0 1 1 0 0],[0 0 1 1 0]);
  wires:
  a/1 -> mapminmax_reverse/1
  mapminmax_reverse/1 -> removeconstantrows_reverse/1
  removeconstantrows_reverse/1 -> y/1

== system hyd_hyb_2_opt_cont_test_new_1_col_ef_fin/hydraulic transmission/PM_hydraulic_machine /eta estimator/eta_t ==
  qv : Inport
  delta_p : Inport  Port=2
  Pmax : Inport  Port=3
  Abs : Abs
  Abs1 : Abs
  Constant : Constant  Value=600
  Constant1 : Constant  Value=0
  Divide : Product  Inputs=*/
  Product : Product  RndMeth=Zero
  Product1 : Product  RndMeth=Zero
  Saturation : Saturate  UpperLimit=1  LowerLimit=0
  Saturation1 : Saturate  UpperLimit=inf  LowerLimit=0.0000001
  Scope : Scope
      settings: SaveName=ScopeData29
  Scope1 : Scope  NumInputPorts=2
      settings: TimeRange=2.2  YMin=-5~-5  YMax=5~5  SaveName=ScopeData30
  Scope2 : Scope
      settings: YMin=0  YMax=190  SaveName=ScopeData50
  Scope3 : Scope
      settings: YMin=0  YMax=190  SaveName=ScopeData51
  Switch : Switch  Threshold=1
  eta_t : Outport
  wires:
  qv/1 -> Product1/1, Abs1/1
  delta_p/1 -> Product1/2
  Pmax/1 -> Product/1
  Constant/1 -> Product/2
  Product1/1 -> Abs/1
  Abs/1 -> Divide/1, Scope1/1
  Product/1 -> Saturation1/1
  Abs1/1 -> Scope2/1, Switch/2
  Saturation/1 -> eta_t/1
  Switch/1 -> Saturation/1, Scope/1
  Divide/1 -> Switch/1, Scope3/1
  Constant1/1 -> Switch/3
  Saturation1/1 -> Divide/2, Scope1/2

== system hyd_hyb_2_opt_cont_test_new_1_col_ef_fin/hydraulic transmission/PM_hydraulic_machine /eta estimator/eta_v ==
  qv : Inport
  vg : Inport  Port=2
  n : Inport  Port=3
  Abs : Abs
  Abs1 : Abs
  Abs2 : Abs
  Constant : Constant  Value=1000
  Constant1 : Constant  Value=0.00001
  Divide : Product  Inputs=*/
  Product : Product  RndMeth=Zero
  Product1 : Product  RndMeth=Zero
  Saturation : Saturate  UpperLimit=1  LowerLimit=0.000001
  Saturation1 : Saturate  UpperLimit=inf  LowerLimit=0.0000001
  Scope : Scope  NumInputPorts=2
      settings: TimeRange=2  YMin=-5~-5  YMax=5~5  SaveName=ScopeData43
  Scope1 : Scope
      settings: TimeRange=2  SaveName=ScopeData44
  Scope2 : Scope  NumInputPorts=2
      settings: TimeRange=2  YMin=-5~-5  YMax=5~5  SaveName=ScopeData45
  Scope3 : Scope  NumInputPorts=2
      settings: TimeRange=2  YMin=-5~-5  YMax=5~5  SaveName=ScopeData46
  Scope4 : Scope
      settings: SaveName=ScopeData52
  Switch : Switch  Threshold=1
  eta_v : Outport
  wires:
  n/1 -> Product/1, Scope2/1
  vg/1 -> Product/2, Scope2/2
  qv/1 -> Scope3/1, Product1/1, Abs2/1
  Constant/1 -> Product1/2
  Product1/1 -> Abs/1
  Abs/1 -> Divide/1, Scope/1
  Product/1 -> Abs1/1
  Abs1/1 -> Scope/2, Saturation1/1
  Divide/1 -> Switch/1, Scope4/1
  Constant1/1 -> Switch/3
  Switch/1 -> Saturation/1, Scope1/1
  Saturation/1 -> eta_v/1
  Abs2/1 -> Switch/2
  Saturation1/1 -> Divide/2

== system hyd_hyb_2_opt_cont_test_new_1_col_ef_fin/hydraulic transmission/accumulator/max - min volume estimator/for 10 gal accumulator ==
  min_press(psi) : Inport
  max_press(psi) : Inport  Port=2
  pre_ch_press(psi) : Inport  Port=3
  Action Port : ActionPort  PropagateVarSize=During execution  ActionType=then
  Constant : Constant  Value=152
  Scope : Scope  NumInputPorts=2
      settings: YMin=-5~-5  YMax=5~5  SaveName=ScopeData40
  Scope1 : Scope  NumInputPorts=2
      settings: YMin=-5~-5  YMax=5~5  SaveName=ScopeData41
  in^3 to lit : Gain  Gain=16.387e-3
  in^3 to lit (1) : Gain  Gain=16.387e-3
  rexroth-1 : Lookup_n-D  BreakpointsForDimension1=[1000,1100,1200,1300,1400,1500,1600,1700,1800,1900,2000,2100,2200,2300,2400,2500,2600,2700,2800,2900,3000,3100,3200,3300,3400,3500,3600,3700,3800,3900,4000,4100,4200,4300,4400,4500,4600,4700,4800,4900,5000,5100,5200,5300,5400,5500,5600,5700,5800,5900,6000]  BreakpointsForDimension2=[1000,1400,2000]  Table=v_p_10  InputSameDT=on
  rexroth-10 : Lookup_n-D  BreakpointsForDimension1=[1000,1100,1200,1300,1400,1500,1600,1700,1800,1900,2000,2100,2200,2300,2400,2500,2600,2700,2800,2900,3000,3100,3200,3300,3400,3500,3600,3700,3800,3900,4000,4100,4200,4300,4400,4500,4600,4700,4800,4900,5000,5100,5200,5300,5400,5500,5600,5700,5800,5900,6000]  BreakpointsForDimension2=[1000,1400,2000]  Table=v_p_10  InputSameDT=on
  min_vol(lit) : Outport
  max_vol(lit) : Outport  Port=2
  accum_dry_mass ( kg ) : Outport  Port=3  InitialOutput=[0]
  wires:
  in^3 to lit/1 -> min_vol(lit)/1, Scope1/1
  rexroth-10/1 -> in^3 to lit (1)/1, Scope/2
  rexroth-1/1 -> in^3 to lit/1, Scope/1
  in^3 to lit (1)/1 -> max_vol(lit)/1, Scope1/2
  pre_ch_press(psi)/1 -> rexroth-10/2, rexroth-1/2
  min_press(psi)/1 -> rexroth-1/1
  max_press(psi)/1 -> rexroth-10/1
  Constant/1 -> accum_dry_mass ( kg )/1

== system hyd_hyb_2_opt_cont_test_new_1_col_ef_fin/hydraulic transmission/accumulator/max - min volume estimator/for 15 gal accumulator1 ==
  min_press(psi) : Inport
  max_press(psi) : Inport  Port=2
  pre_ch_press(psi) : Inport  Port=3
  Action Port : ActionPort  PropagateVarSize=During execution  ActionType=then
  Constant : Constant  Value=220
  Scope : Scope  NumInputPorts=2
      settings: YMin=-5~-5  YMax=5~5  SaveName=ScopeData38
  Scope1 : Scope  NumInputPorts=2
      settings: YMin=4.74484~24.0403  YMax=4.74484~24.0403  SaveName=ScopeData39
  in^3 to lit : Gain  Gain=16.387e-3
  in^3 to lit (1) : Gain  Gain=16.387e-3
  rexroth-1 : Lookup_n-D  BreakpointsForDimension1=[1000,1100,1200,1300,1400,1500,1600,1700,1800,1900,2000,2100,2200,2300,2400,2500,2600,2700,2800,2900,3000,3100,3200,3300,3400,3500,3600,3700,3800,3900,4000,4100,4200,4300,4400,4500,4600,4700,4800,4900,5000,5100,5200,5300,5400,5500,5600,5700,5800,5900,6000]  BreakpointsForDimension2=[1000,1400,2000]  Table=v_p_15  InputSameDT=on
  rexroth-15 : Lookup_n-D  BreakpointsForDimension1=[1000,1100,1200,1300,1400,1500,1600,1700,1800,1900,2000,2100,2200,2300,2400,2500,2600,2700,2800,2900,3000,3100,3200,3300,3400,3500,3600,3700,3800,3900,4000,4100,4200,4300,4400,4500,4600,4700,4800,4900,5000,5100,5200,5300,5400,5500,5600,5700,5800,5900,6000]  BreakpointsForDimension2=[1000,1400,2000]  Table=v_p_15  InputSameDT=on
  min_vol(lit) : Outport
  max_vol(lit) : Outport  Port=2
  accum_dry_mass ( kg ) : Outport  Port=3  InitialOutput=[0]
  wires:
  in^3 to lit/1 -> min_vol(lit)/1, Scope1/1
  rexroth-1/1 -> in^3 to lit (1)/1, Scope/2
  rexroth-15/1 -> in^3 to lit/1, Scope/1
  in^3 to lit (1)/1 -> max_vol(lit)/1, Scope1/2
  pre_ch_press(psi)/1 -> rexroth-15/2, rexroth-1/2
  min_press(psi)/1 -> rexroth-15/1
  max_press(psi)/1 -> rexroth-1/1
  Constant/1 -> accum_dry_mass ( kg )/1

== system hyd_hyb_2_opt_cont_test_new_1_col_ef_fin/hydraulic transmission/accumulator/max - min volume estimator/for 5 gal accumulator ==
  min_press(psi) : Inport
  max_press(psi) : Inport  Port=2
  pre_ch_press(psi) : Inport  Port=3
  Action Port : ActionPort  PropagateVarSize=During execution  ActionType=then
  Constant : Constant  Value=100
  Scope : Scope  NumInputPorts=2
      settings: YMin=-5~-5  YMax=5~5  SaveName=ScopeData27
  Scope1 : Scope  NumInputPorts=2
      settings: YMin=61.8714~626.852  YMax=61.8714~626.852  SaveName=ScopeData28
  in^3 to lit : Gain  Gain=16.387e-3
  in^3 to lit (1) : Gain  Gain=16.387e-3
  rexroth-1 : Lookup_n-D  BreakpointsForDimension1=[1000,1100,1200,1300,1400,1500,1600,1700,1800,1900,2000,2100,2200,2300,2400,2500,2600,2700,2800,2900,3000,3100,3200,3300,3400,3500,3600,3700,3800,3900,4000,4100,4200,4300,4400,4500,4600,4700,4800,4900,5000,5100,5200,5300,5400,5500,5600,5700,5800,5900,6000]  BreakpointsForDimension2=[1000,1400,2000]  Table=v_p_5  InputSameDT=on
  rexroth-5 : Lookup_n-D  BreakpointsForDimension1=[1000,1100,1200,1300,1400,1500,1600,1700,1800,1900,2000,2100,2200,2300,2400,2500,2600,2700,2800,2900,3000,3100,3200,3300,3400,3500,3600,3700,3800,3900,4000,4100,4200,4300,4400,4500,4600,4700,4800,4900,5000,5100,5200,5300,5400,5500,5600,5700,5800,5900,6000]  BreakpointsForDimension2=[1000,1400,2000]  Table=v_p_5  InputSameDT=on
  min_vol(lit) : Outport
  max_vol(lit) : Outport  Port=2
  accum_dry_mass ( kg ) : Outport  Port=3  InitialOutput=[0]
  wires:
  in^3 to lit/1 -> min_vol(lit)/1, Scope/1
  rexroth-1/1 -> in^3 to lit (1)/1, Scope1/2
  rexroth-5/1 -> in^3 to lit/1, Scope1/1
  in^3 to lit (1)/1 -> max_vol(lit)/1, Scope/2
  pre_ch_press(psi)/1 -> rexroth-5/2, rexroth-1/2
  min_press(psi)/1 -> rexroth-5/1
  max_press(psi)/1 -> rexroth-1/1
  Constant/1 -> accum_dry_mass ( kg )/1

== system hyd_hyb_2_opt_cont_test_new_1_col_ef_fin/Transmission1/Torque Convertor/main solver/Sensor(TC_in)/Motion sensor ==
  Ideal Rotational Motion Sensor : fl_lib/Mechanical/Mechanical Sensors/Ideal Rotational Motion Sensor  SystemSampleTime=-1  offset=0 rad  w_Log=off  t_Log=off  phi_Log=off  LocalVarNames=|w|t|phi  LocalVarDescs=|w|t|phi  LocalVarLogging=[]
  MRR : fl_lib/Mechanical/Rotational Elements/Mechanical Rotational Reference  SystemSampleTime=-1  t_Log=off  LocalVarNames=|t  LocalVarDescs=|t  LocalVarLogging=[]
  PS-Simulink Converter : nesl_utility/PS-Simulink Converter  SystemSampleTime=-1  PhysicalDomain=network_engine_domain  LeftPortType=input  RightPortType=output  SubClassName=ps_output  Unit=rad/s  AffineConversion=off
  A : PMIOPort  Port=1  Side=Left
  W : Outport
  wires:
  PS-Simulink Converter/1 -> W/1
  connections:
  A/RConn1 -- Ideal Rotational Motion Sensor/LConn1
  Ideal Rotational Motion Sensor/RConn2 -- PS-Simulink Converter/LConn1
  MRR/LConn1 -- Ideal Rotational Motion Sensor/RConn1

== system hyd_hyb_2_opt_cont_test_new_1_col_ef_fin/Transmission1/Torque Convertor/main solver/Sensor(TC_in)/Torque sensor ==
  PS2S : nesl_utility/PS-Simulink Converter  SystemSampleTime=-1  PhysicalDomain=network_engine_domain  LeftPortType=input  RightPortType=output  SubClassName=ps_output  Unit=1  AffineConversion=off
  Torque Sensor : fl_lib/Mechanical/Mechanical Sensors/Ideal Torque Sensor  SystemSampleTime=-1  w_Log=off  t_Log=off  LocalVarNames=|w|t  LocalVarDescs=|w|t  LocalVarLogging=[]
  B : PMIOPort  Port=1  Side=Right
  A : PMIOPort  Port=2  Side=Left
  T : Outport
  wires:
  PS2S/1 -> T/1
  connections:
  A/RConn1 -- Torque Sensor/LConn1
  B/RConn1 -- Torque Sensor/RConn1
  Torque Sensor/RConn2 -- PS2S/LConn1
